simulink model "scheme_sim"  (R2020b)
settings: Solver=ode23t  StartTime=0.0  StopTime=5  RelTol=1e-3
values from neighbouring files (symbols this model uses):
  Kd = 3e2*eye(3)    [init_simulink.m]    (also in plotFig.m)
  Kp = 1e6*eye(3)    [init_simulink.m]    (also in plotFig.m)
  qt = qt+([q(1:2,1);50*q(3,1)]'-[qt(1,1:2),qt(1,3)])    [Ident_model.m]    (also in plotFig.m)
settings Model: Creator=Administrator  LastModifiedBy=maxjo
settings DataIOCC: SaveFormat=Array  SaveOutput=off  SignalLogging=off  DSMLogging=off  SaveTime=off  ReturnWorkspaceOutputs=off

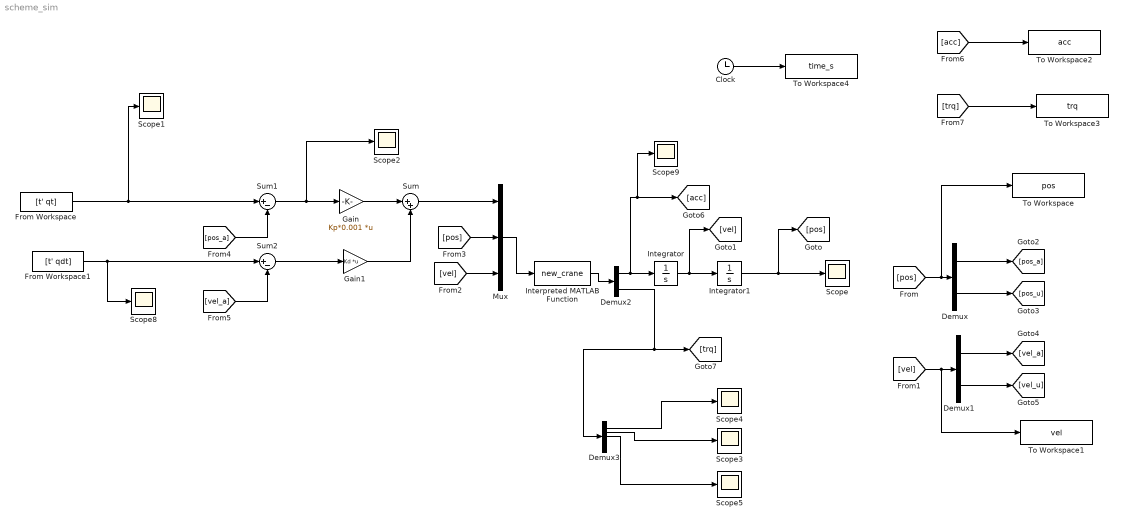
== system scheme_sim ==
  Clock : Clock
  Demux : Demux  Outputs=[3 2]
  Demux1 : Demux  Outputs=[3 2]
  Demux2 : Demux  Outputs=[5 5]
  Demux3 : Demux  Outputs=5
  From Workspace : FromWorkspace  VariableName=[t' qt]
  From Workspace1 : FromWorkspace  VariableName=[t' qdt]
  Gain : Gain  Gain=Kp*0.001  Multiplication=Matrix(K*u)
  Gain1 : Gain  Gain=Kd  Multiplication=Matrix(K*u)
  Integrator : Integrator  InitialCondition=[0 0 0 0 0]
  Integrator1 : Integrator  InitialCondition=[qt(1,:)';0;0]
  Interpreted MATLAB Function : MATLABFcn  MATLABFcn=new_crane
  Mux : Mux  Inputs=[3 5 5]
  Scope{,1..5,8..9} (8 alike) : Scope
  Sum : Sum  Inputs=|++
  Sum1 : Sum  Inputs=|+-
  Sum2 : Sum  Inputs=|+-
  To Workspace : ToWorkspace  VariableName=pos  SampleTime=-1
  To Workspace1 : ToWorkspace  VariableName=vel  SampleTime=-1
  To Workspace2 : ToWorkspace  VariableName=acc  SampleTime=-1
  To Workspace3 : ToWorkspace  VariableName=trq  SampleTime=-1
  To Workspace4 : ToWorkspace  VariableName=time_s  SampleTime=-1
  wires:
  Integrator/1 -> [vel], Integrator1/1
  Mux/1 -> Interpreted MATLAB Function/1
  Integrator1/1 -> [pos], Scope/1
  Sum/1 -> Mux/1
  Gain/1 -> Sum/1
  Gain1/1 -> Sum/2
  Sum1/1 -> Scope2/1, Gain/1
  Sum2/1 -> Gain1/1
  [pos] -> To Workspace/1, Demux/1
  [vel] -> To Workspace1/1, Demux1/1
  Demux/1 -> [pos_a]
  Demux/2 -> [pos_u]
  Demux1/1 -> [vel_a]
  Demux1/2 -> [vel_u]
  [vel] -> Mux/3
  [pos] -> Mux/2
  [pos_a] -> Sum1/2
  [vel_a] -> Sum2/2
  From Workspace/1 -> Scope1/1, Sum1/1
  From Workspace1/1 -> Scope8/1, Sum2/1
  Interpreted MATLAB Function/1 -> Demux2/1
  Demux2/1 -> Scope9/1, [acc], Integrator/1
  Demux2/2 -> [trq], Demux3/1
  [acc] -> To Workspace2/1
  [trq] -> To Workspace3/1
  Clock/1 -> To Workspace4/1
  Demux3/1 -> Scope4/1
  Demux3/2 -> Scope3/1
  Demux3/3 -> Scope5/1
